simulink model "Stirred_tank_heater_PI_Control"  (R2017b)
settings: Solver=VariableStepAuto  StartTime=0.0  StopTime=4  RelTol=1e-3
settings Model: Creator=HP  LastModifiedBy=HP

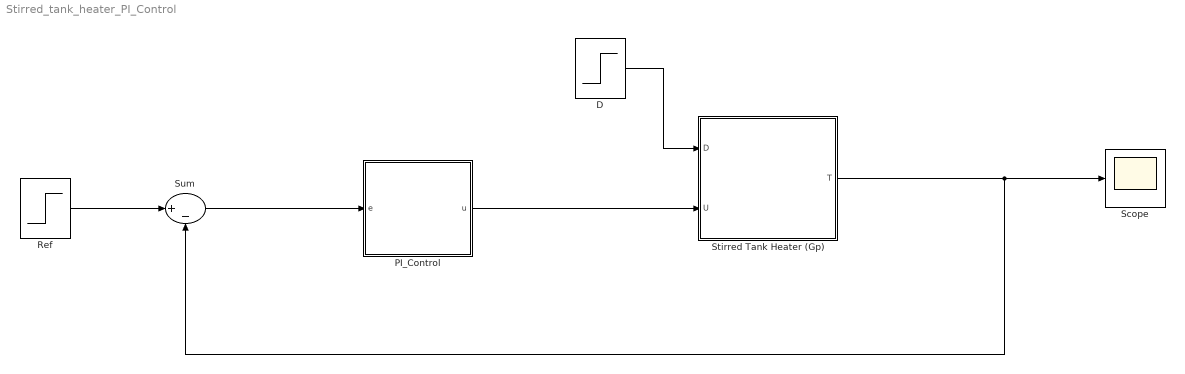
== system Stirred_tank_heater_PI_Control ==
  D : Step  Time=2  After=0  SampleTime=0.01
  PI_Control : Subsystem
  Ref : Step  Time=0  SampleTime=0.01
  Scope : Scope
  Stirred Tank Heater (Gp) : Subsystem
  Sum : Sum  Inputs=|+-
  wires:
  Stirred Tank Heater (Gp)/1(T) -> Scope/1, Sum/2
  Ref/1 -> Sum/1
  D/1 -> Stirred Tank Heater (Gp)/1(D)
  PI_Control/1(u) -> Stirred Tank Heater (Gp)/2(U)
  Sum/1 -> PI_Control/1(e)

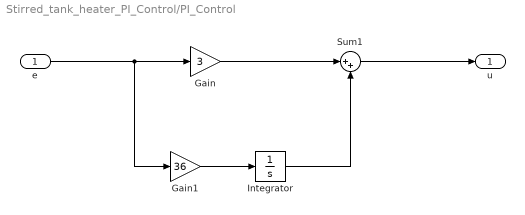
== system Stirred_tank_heater_PI_Control/PI_Control ==
  e : Inport
  Gain : Gain  Gain=3
  Gain1 : Gain  Gain=36
  Integrator : Integrator
  Sum1 : Sum  Inputs=|++
  u : Outport
  wires:
  Gain/1 -> Sum1/1
  Sum1/1 -> u/1
  e/1 -> Gain1/1, Gain/1
  Integrator/1 -> Sum1/2
  Gain1/1 -> Integrator/1

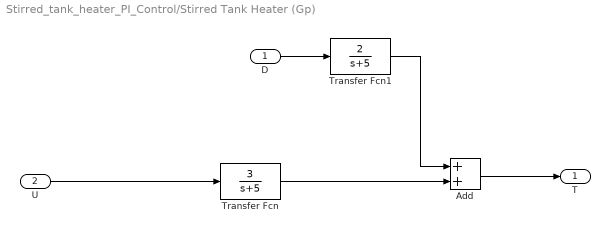
== system Stirred_tank_heater_PI_Control/Stirred Tank Heater (Gp) ==
  D : Inport
  U : Inport  Port=2
  Add : Sum
  Transfer Fcn : TransferFcn  Numerator=[3]  Denominator=[1 5]
  Transfer Fcn1 : TransferFcn  Numerator=[2]  Denominator=[1 5]
  T : Outport
  wires:
  U/1 -> Transfer Fcn/1
  Add/1 -> T/1
  Transfer Fcn/1 -> Add/2
  Transfer Fcn1/1 -> Add/1
  D/1 -> Transfer Fcn1/1
